simulink model "eight"  (R2020b)
settings: Solver=VariableStepAuto  StartTime=0.0  StopTime=10.0  RelTol=1e-3
settings Model: Creator=Dell  LastModifiedBy=VIVEK

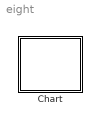
== system eight ==
  Chart : Stateflow chart  TreatAsAtomicUnit=on

== stateflow chart eight/Chart ==
  state y = FloorCheck(Floor) [function]
    (default) -> (junction 33)
    (junction 33) -> (junction 29) [order 3] : [FloorSelect<Floor]{
        | send(down);
        | disp('LiftMovingDown');}
    (junction 33) -> (junction 34) [order 1] : [FloorSelect>Floor]{
        | send(up);
        | disp('LiftMovingUp');}
    (junction 29) -> (junction 30)
    (junction 33) -> (junction 26) [order 2] : [FloorSelect==Floor]{
        | disp('CurrentFloor');}
    (junction 34) -> (junction 31)
    (junction 30) -> (junction 26)
    (junction 31) -> (junction 26)
    (junction 26) -> (junction 32)
  data: Floor function_input; y function_output
